simulink subsystem "calc_vec_angle"  (R2021a)
settings: Solver=VariableStepAuto  StartTime=0.0  StopTime=10.0  RelTol=1e-3
settings Model: Creator=EpEp  LastModifiedBy=EpEp

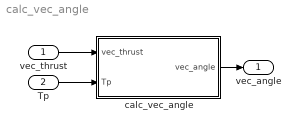
== system calc_vec_angle ==
  vec_thrust : Inport
  Tp : Inport  Port=2
  calc_vec_angle : MATLAB Function  TreatAsAtomicUnit=on
  vec_angle : Outport
  wires:
  vec_thrust/1 -> calc_vec_angle/1(vec_thrust)
  Tp/1 -> calc_vec_angle/2(Tp)
  calc_vec_angle/1(vec_angle) -> vec_angle/1

== matlab function calc_vec_angle/calc_vec_angle ==
  data: vec_thrust input; vec_angle output; Tp input
function vec_angle = fcn(vec_thrust, Tp)
    if abs(vec_thrust) >= Tp
        vec_angle = pi;
    else
        vec_angle = asin(vec_thrust/Tp);
    end
